simulink model "control"  (R2021a)
settings: Solver=VariableStepAuto  StartTime=0.0  StopTime=10  RelTol=1e-3
libraries: dsparch4 x1
settings Model: Creator=Abdullah All Noman  LastModifiedBy=Abdullah All Noman

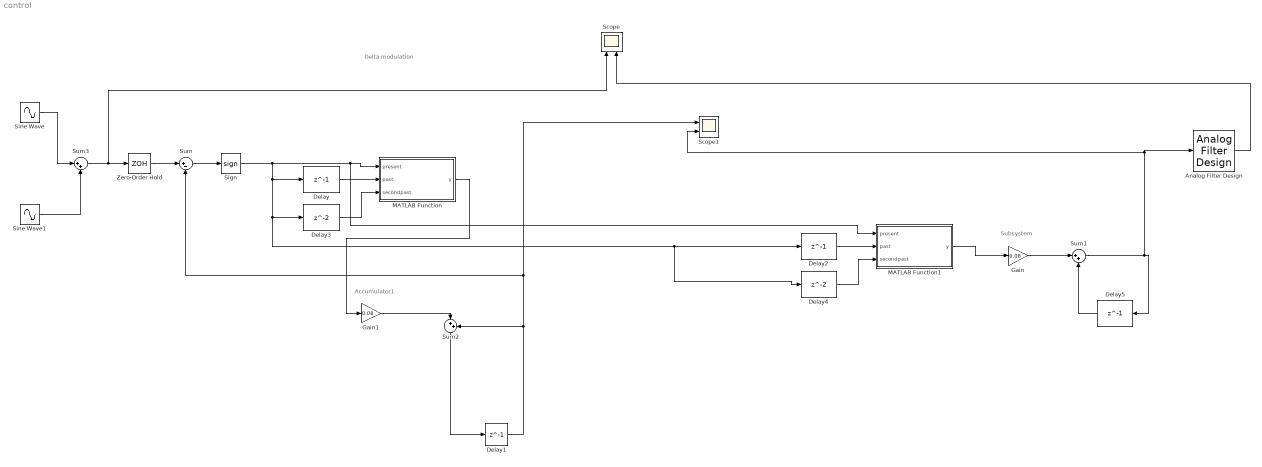
== system control ==
  note: Subsystem
  note: Delta modulation
  note: Accumulator1
  Analog Filter Design : dsparch4/Analog Filter Design  method=Butterworth  filttype=Lowpass  N=8  Wlo=2*pi*400  Whi=80  Rp=2  Rs=40
  Delay : Delay  DelayLength=1  InputProcessing=Columns as channels (frame based)
  Delay1 : Delay  DelayLength=1
  Delay2 : Delay  DelayLength=1  InputProcessing=Columns as channels (frame based)
  Delay3 : Delay  InputProcessing=Columns as channels (frame based)
  Delay4 : Delay  InputProcessing=Columns as channels (frame based)
  Delay5 : Delay  DelayLength=1  InputProcessing=Columns as channels (frame based)
  Gain : Gain  Gain=0.08
  Gain1 : Gain  Gain=0.08
  MATLAB Function : MATLAB Function  TreatAsAtomicUnit=on
  MATLAB Function1 : MATLAB Function  TreatAsAtomicUnit=on
  Scope : Scope  NumInputPorts=2
  Scope1 : Scope  NumInputPorts=2
  Sign : Signum
  Sine Wave : Sin  Frequency=2*pi*100  SampleTime=0
  Sine Wave1 : Sin  Frequency=2*pi*300  SampleTime=0
  Sum : Sum  Inputs=|+-
  Sum1 : Sum  Inputs=|++
  Sum2 : Sum  Inputs=|++
  Sum3 : Sum  Inputs=|++
  Zero-Order Hold : ZeroOrderHold  SampleTime=1/16000
  wires:
  Delay1/1 -> Sum2/2, Scope1/1, Sum/2
  Sum2/1 -> Delay1/1
  Zero-Order Hold/1 -> Sum/1
  Gain1/1 -> Sum2/1
  Sum3/1 -> Scope/1, Zero-Order Hold/1
  Sum/1 -> Sign/1
  Sine Wave/1 -> Sum3/1
  Sine Wave1/1 -> Sum3/2
  Delay/1 -> MATLAB Function/2(past)
  Delay3/1 -> MATLAB Function/3(secondpast)
  MATLAB Function/1(y) -> Gain1/1
  Analog Filter Design/1 -> Scope/2
  Sign/1 -> Delay4/1, Delay2/1, Delay3/1, Delay/1, MATLAB Function1/1(present), MATLAB Function/1(present)
  Delay4/1 -> MATLAB Function1/3(secondpast)
  Delay2/1 -> MATLAB Function1/2(past)
  Sum1/1 -> Analog Filter Design/1, Scope1/2, Delay5/1
  MATLAB Function1/1(y) -> Gain/1
  Delay5/1 -> Sum1/2
  Gain/1 -> Sum1/1

== matlab function control/MATLAB Function ==
  data: present input; y output; past input; secondpast input
function y = control(present,past,secondpast)

if present == past 
    if present == secondpast
        y=4*present;
    else
        y=2*present;
    end
else
    y=1*present;
    
end
end

== matlab function control/MATLAB Function1 ==
  data: present input; y output; past input; secondpast input
function y = control(present,past,secondpast)

if present == past 
    if present == secondpast
        y=4*present;
    else
        y=2*present;
    end
else
    y=1*present;
    
end
end
